simulink model "Message_eg2"  (R2018a)
settings: Solver=VariableStepAuto  StartTime=0.0  StopTime=10.0  RelTol=1e-3
settings Model: Creator=86188  LastModifiedBy=86188

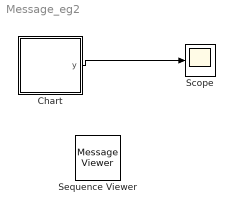
== system Message_eg2 ==
  Chart : Stateflow chart  TreatAsAtomicUnit=on
  Scope : Scope
  Sequence Viewer : MessageViewer
  wires:
  Chart/1(y) -> Scope/1

== stateflow chart Message_eg2/Chart ==
  state A
    en:
    M.data=3;
    M1.data=4;
    send(M);
    send(M1);
  state B
    y=1;
  (default) -> A
  A -> B : M[M1.data==4]
  data: M local; y output; M1 local
